simulink model "limit"  (R2014b)
settings: Solver=ode45  StartTime=0.0  StopTime=100  RelTol=1e-3
undefined symbols (not defined in the file or in its folder): Fc, Fs, Ki, Kp, Kv, m, sigma0, sigma1, sigma2, vs
settings Model: CovSFcnEnable=on  Creator=hank  LastModifiedBy=123
settings OptimizationCC: UseDivisionForNetSlopeComputation=off  SimCompilerOptimization=off
settings DebuggingCC: SolverPrmCheckMsg=none  FrameProcessingCompatibilityMsg=error
settings RTWCC: RTWCompilerOptimization=off

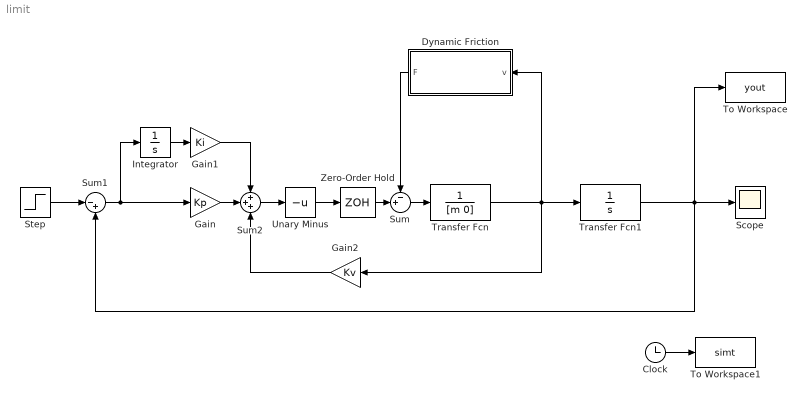
== system limit ==
  Clock : Clock
  Dynamic Friction : Subsystem
      mask Display:
      | text(32,30,'Dynamic')
      | text(35,15,'Friction')
  Gain : Gain  Gain=Kp
  Gain1 : Gain  Gain=Ki
  Gain2 : Gain  Gain=Kv
  Integrator : Integrator
  Scope : Scope
      settings: TickLabels=on  ShowLegends=on  YMin=-8.41871e-44  YMax=2  ScrollMode=on
  Step : Step  Time=0  SampleTime=0
  Sum : Sum  Inputs=-+|
  Sum1 : Sum  Inputs=|-+
  Sum2 : Sum  Inputs=+++
  To Workspace : ToWorkspace  VariableName=yout  SampleTime=-1
  To Workspace1 : ToWorkspace  VariableName=simt  SampleTime=-1
  Transfer Fcn : TransferFcn  Denominator=[m 0]
  Transfer Fcn1 : TransferFcn  Denominator=[1 0]
  Unary Minus : UnaryMinus
  Zero-Order Hold : ZeroOrderHold  SampleTime=5e-5
  wires:
  Transfer Fcn/1 -> Dynamic Friction/1(v), Gain2/1, Transfer Fcn1/1
  Sum/1 -> Transfer Fcn/1
  Dynamic Friction/1(F) -> Sum/1
  Transfer Fcn1/1 -> Scope/1, To Workspace/1, Sum1/2
  Step/1 -> Sum1/1
  Sum1/1 -> Integrator/1, Gain/1
  Integrator/1 -> Gain1/1
  Gain2/1 -> Sum2/3
  Gain1/1 -> Sum2/1
  Gain/1 -> Sum2/2
  Clock/1 -> To Workspace1/1
  Unary Minus/1 -> Zero-Order Hold/1
  Sum2/1 -> Unary Minus/1
  Zero-Order Hold/1 -> Sum/2

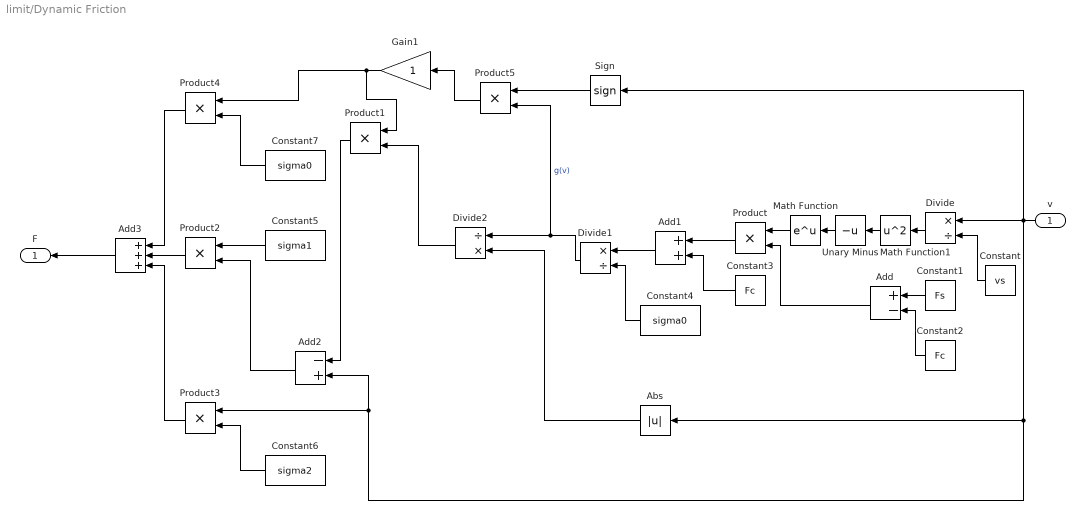
== system limit/Dynamic Friction ==
  v : Inport
  Abs : Abs  ZeroCross=off
  Add : Sum  Inputs=+-
  Add1 : Sum
  Add2 : Sum  Inputs=-+
  Add3 : Sum  Inputs=+++
  Constant : Constant  Value=vs
  Constant1 : Constant  Value=Fs
  Constant2 : Constant  Value=Fc
  Constant3 : Constant  Value=Fc
  Constant4 : Constant  Value=sigma0
  Constant5 : Constant  Value=sigma1
  Constant6 : Constant  Value=sigma2
  Constant7 : Constant  Value=sigma0
  Divide : Product  Inputs=*/
  Divide1 : Product  Inputs=*/
  Divide2 : Product  Inputs=/*
  Gain1 : Gain
  Math Function : Math  SaturateOnIntegerOverflow=on
  Math Function1 : Math  Operator=square  SaturateOnIntegerOverflow=on
  Product{,1..5} (6 alike) : Product
  Sign : Signum  ZeroCross=off
  Unary Minus : UnaryMinus
  F : Outport
  wires:
  v/1 -> Sign/1, Abs/1, Add2/2, Product3/1, Divide/1
  Constant/1 -> Divide/2
  Constant1/1 -> Add/1
  Constant2/1 -> Add/2
  Add/1 -> Product/2
  Product/1 -> Add1/1
  Constant3/1 -> Add1/2
  Add1/1 -> Divide1/1
  Constant4/1 -> Divide1/2
  Product1/1 -> Add2/1
  Add2/1 -> Product2/2
  Constant5/1 -> Product2/1
  Constant6/1 -> Product3/2
  Constant7/1 -> Product4/2
  Product2/1 -> Add3/2
  Product3/1 -> Add3/3
  Product4/1 -> Add3/1
  Add3/1 -> F/1
  Divide/1 -> Math Function1/1
  Math Function1/1 -> Unary Minus/1
  Math Function/1 -> Product/1
  Unary Minus/1 -> Math Function/1
  Divide1/1 -> Product5/2, Divide2/1  "g(v)"
  Abs/1 -> Divide2/2
  Sign/1 -> Product5/1
  Divide2/1 -> Product1/2
  Product5/1 -> Gain1/1
  Gain1/1 -> Product1/1, Product4/1
